simulink model "tiny_sl_model"  (Simulink 6.6)
settings: Solver=FixedStepDiscrete  StartTime=0.0  StopTime=10.0  FixedStep=1  RelTol=1e-3
settings Model: Creator=Administrator  LastModifiedBy=Administrator

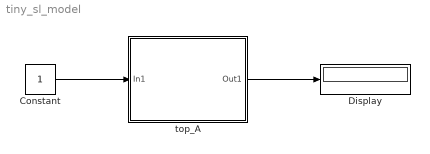
== system tiny_sl_model ==
  Constant : Constant
  Display : Display
  top_A : Subsystem
  wires:
  top_A/1(Out1) -> Display/1
  Constant/1 -> top_A/1(In1)

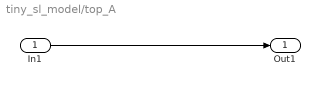
== system tiny_sl_model/top_A ==
  In1 : Inport
  Out1 : Outport
  wires:
  In1/1 -> Out1/1
